simulink model "vending_melay"  (R2020a)
settings: Solver=VariableStepAuto  StartTime=0.0  StopTime=200  RelTol=1e-3
settings Model: Creator=Shubham  LastModifiedBy=Shubham

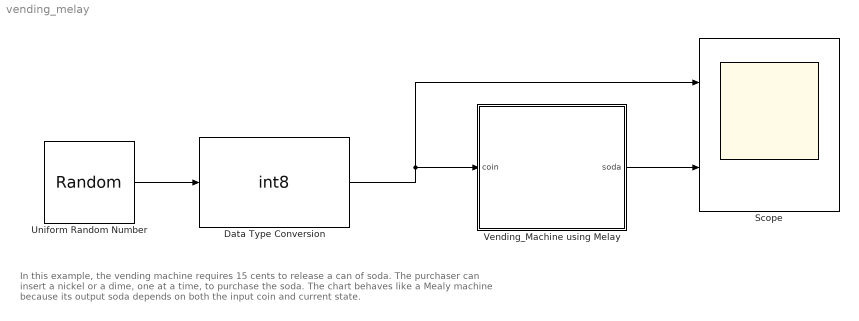
== system vending_melay ==
  note: In this example, the vending machine requires 15 cents to release a can of soda.
      | The purchaser can insert a nickel or a dime, one at a time, to purchase the soda.
      | The chart behaves like a Mealy machine because its output soda depends on both the input coin and current state.
  Data Type Conversion : DataTypeConversion  OutDataTypeStr=int8  RndMeth=Nearest  SaturateOnIntegerOverflow=on
  Scope : Scope  NumInputPorts=2
  Uniform Random Number : UniformRandomNumber  Minimum=0  Maximum=2  Seed=337  SampleTime=10
  Vending_Machine using Melay : Stateflow chart  TreatAsAtomicUnit=on
  wires:
  Data Type Conversion/1 -> Scope/1, Vending_Machine using Melay/1(coin)
  Uniform Random Number/1 -> Data Type Conversion/1
  Vending_Machine using Melay/1(soda) -> Scope/2

== stateflow chart vending_melay/Vending_Machine using Melay ==
  state got_0
  state got_nickel
  state got_dime
  (default) -> got_0
  got_0 -> got_nickel [order 1] : [coin==1]{soda=0}
  got_nickel -> got_0 [order 2] : [coin==2]{soda=1}
  got_nickel -> got_dime [order 1] : [coin==1]{soda=0}
  got_dime -> got_nickel [order 2] : [coin==2]{soda=1}
  got_dime -> got_0 [order 1] : [coin==1]{soda=1}
  got_0 -> got_dime [order 2] : [coin==2]{soda=0}
  data: coin input; soda output
